simulink model "Wheelspeed"  (R2015b)
settings: Solver=FixedStepAuto  StartTime=0.0  StopTime=100.0  RelTol=1e-3
libraries: simulink x4, arduinolib x4
settings Model: SimulationMode=external  ExtModeTrigDuration=2  Creator=Joern  LastModifiedBy=Joern
settings OptimizationCC: OptimizeModelRefInitCode=on  LifeSpan=1  MaxStackSize=64
settings HardwareCC: ProdBitPerInt=16  ProdBitPerPointer=16  ProdLargestAtomicFloat=None  ProdWordSize=8  ProdHWDeviceType=Atmel->AVR
settings RTWCC: SystemTargetFile=ert.tlc  TemplateMakefile=ert_default_tmf  Description=Embedded Coder  Toolchain=Arduino AVR v1.6.1  BuildConfiguration=Faster Runs
settings CodeAppCC: IgnoreCustomStorageClasses=off
settings ERTTargetCC: GenerateSampleERTMain=on  SupportContinuousTime=on  SupportVariableSizeSignals=on

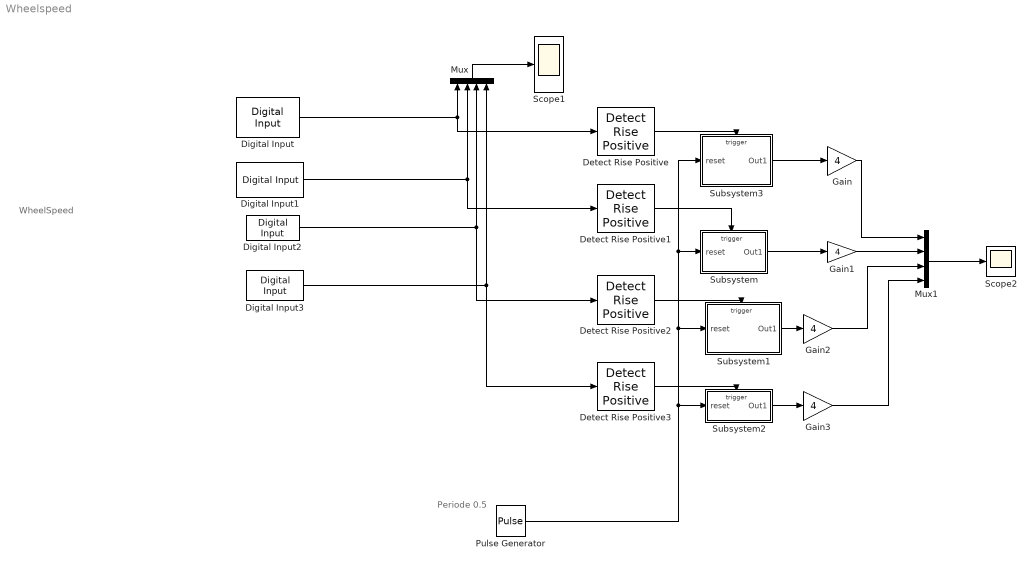
== system Wheelspeed ==
  note: Periode 0.5
  note: WheelSpeed
  Detect Rise Positive{,1..3} (4 alike) : simulink/Logic and Bit Operations/Detect Rise Positive  vinit=0  InputProcessing=Inherited  OutDataTypeStr=boolean
  Digital Input : arduinolib/Digital Input  pinNumber=18  sampleTime=0.01  blockPlatform=arduino
  Digital Input1 : arduinolib/Digital Input  pinNumber=19  sampleTime=0.01  blockPlatform=arduino
  Digital Input2 : arduinolib/Digital Input  pinNumber=2  sampleTime=0.01  blockPlatform=arduino
  Digital Input3 : arduinolib/Digital Input  pinNumber=3  sampleTime=0.01  blockPlatform=arduino
  Gain{,1..3} (4 alike) : Gain  Gain=4
  Mux : Mux
  Mux1 : Mux
  Pulse Generator : DiscretePulseGenerator  PulseType=Time based  Period=0.5
  Scope1 : Scope
  Scope2 : Scope
  Subsystem : Subsystem
  Subsystem1 : Subsystem
  Subsystem2 : Subsystem
  Subsystem3 : Subsystem
  wires:
  Mux/1 -> Scope1/1
  Digital Input/1 -> Detect Rise Positive/1, Mux/1
  Digital Input1/1 -> Mux/2, Detect Rise Positive1/1
  Digital Input2/1 -> Mux/3, Detect Rise Positive2/1
  Digital Input3/1 -> Mux/4, Detect Rise Positive3/1
  Detect Rise Positive/1 -> Subsystem3/Trigger
  Detect Rise Positive1/1 -> Subsystem/Trigger
  Detect Rise Positive2/1 -> Subsystem1/Trigger
  Detect Rise Positive3/1 -> Subsystem2/Trigger
  Subsystem3/1(Out1) -> Gain/1
  Subsystem/1(Out1) -> Gain1/1
  Subsystem1/1(Out1) -> Gain2/1
  Subsystem2/1(Out1) -> Gain3/1
  Mux1/1 -> Scope2/1
  Pulse Generator/1 -> Subsystem2/1(reset), Subsystem1/1(reset), Subsystem/1(reset), Subsystem3/1(reset)
  Gain/1 -> Mux1/1
  Gain1/1 -> Mux1/2
  Gain2/1 -> Mux1/3
  Gain3/1 -> Mux1/4

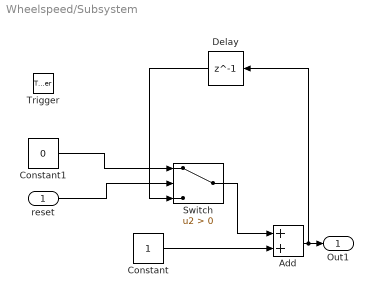
== system Wheelspeed/Subsystem ==
  reset : Inport
  Trigger : TriggerPort  PortDimensions=1
  Add : Sum  Inputs=2
  Constant : Constant
  Constant1 : Constant  Value=0
  Delay : Delay  DelayLength=1  InitialCondition=0
  Switch : Switch  Criteria=u2 > Threshold
  Out1 : Outport
  wires:
  Add/1 -> Delay/1, Out1/1
  Constant/1 -> Add/2
  reset/1 -> Switch/2
  Constant1/1 -> Switch/1
  Switch/1 -> Add/1
  Delay/1 -> Switch/3

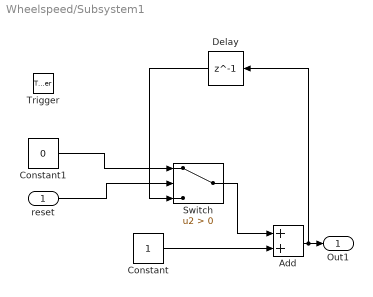
== system Wheelspeed/Subsystem1 ==
  reset : Inport
  Trigger : TriggerPort  PortDimensions=1
  Add : Sum  Inputs=2
  Constant : Constant
  Constant1 : Constant  Value=0
  Delay : Delay  DelayLength=1  InitialCondition=0
  Switch : Switch  Criteria=u2 > Threshold
  Out1 : Outport
  wires:
  Delay/1 -> Switch/3
  Switch/1 -> Add/1
  Constant1/1 -> Switch/1
  reset/1 -> Switch/2
  Constant/1 -> Add/2
  Add/1 -> Out1/1, Delay/1

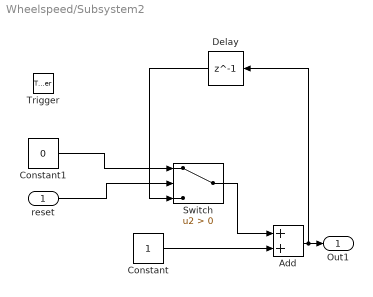
== system Wheelspeed/Subsystem2 ==
  reset : Inport
  Trigger : TriggerPort  PortDimensions=1
  Add : Sum  Inputs=2
  Constant : Constant
  Constant1 : Constant  Value=0
  Delay : Delay  DelayLength=1  InitialCondition=0
  Switch : Switch  Criteria=u2 > Threshold
  Out1 : Outport
  wires:
  Add/1 -> Delay/1, Out1/1
  Constant/1 -> Add/2
  reset/1 -> Switch/2
  Constant1/1 -> Switch/1
  Switch/1 -> Add/1
  Delay/1 -> Switch/3

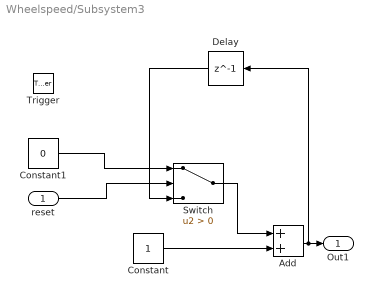
== system Wheelspeed/Subsystem3 ==
  reset : Inport
  Trigger : TriggerPort  PortDimensions=1
  Add : Sum  Inputs=2
  Constant : Constant
  Constant1 : Constant  Value=0
  Delay : Delay  DelayLength=1  InitialCondition=0
  Switch : Switch  Criteria=u2 > Threshold
  Out1 : Outport
  wires:
  Delay/1 -> Switch/3
  Switch/1 -> Add/1
  Constant1/1 -> Switch/1
  reset/1 -> Switch/2
  Constant/1 -> Add/2
  Add/1 -> Out1/1, Delay/1
